simulink model "ejemplo_pendulo"  (R2018a)
settings: Solver=VariableStepAuto  StartTime=0.0  StopTime=4  MaxStep=1e-2  RelTol=1e-3
InitFcn:
  | simulacion
values from neighbouring files (symbols this model uses):
  Xe = [0 0]    [simulacion_pendulo.m]
  Xini = [0.8 0]    [simulacion_pendulo.m]
  Xinil = Xini-Xe    [simulacion_pendulo.m]
libraries: simulink x1
settings Model: Creator=cmparedes  LastModifiedBy=carma

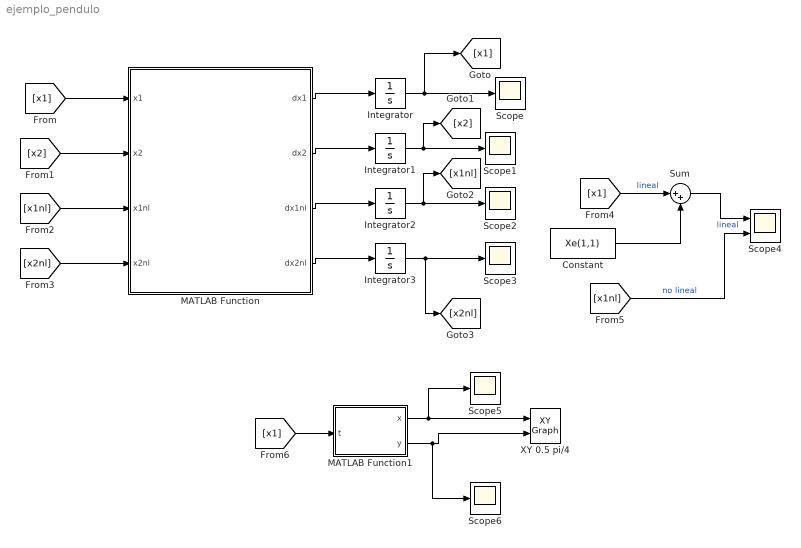
== system ejemplo_pendulo ==
  Constant : Constant  Value=Xe(1,1)
  Integrator : Integrator  InitialCondition=Xinil(1,1)
  Integrator1 : Integrator  InitialCondition=Xinil(1,2)
  Integrator2 : Integrator  InitialCondition=Xini(1,1)
  Integrator3 : Integrator  InitialCondition=Xini(1,2)
  MATLAB Function : MATLAB Function  TreatAsAtomicUnit=on
  MATLAB Function1 : MATLAB Function  TreatAsAtomicUnit=on
  Scope{,1..3,5..6} (6 alike) : Scope
  Scope4 : Scope  NumInputPorts=2
  Sum : Sum  Inputs=|++
  XY 0.5 pi/4 : simulink/Sinks/XY Graph  xmin=-0.5  xmax=0.45  ymin=-1.01  ymax=-0.92  st=-1
  wires:
  MATLAB Function/1(dx1) -> Integrator/1
  MATLAB Function/2(dx2) -> Integrator1/1
  MATLAB Function/3(dx1nl) -> Integrator2/1
  MATLAB Function/4(dx2nl) -> Integrator3/1
  Integrator/1 -> [x1], Scope/1
  Integrator1/1 -> [x2], Scope1/1
  Integrator2/1 -> [x1nl], Scope2/1
  Integrator3/1 -> [x2nl], Scope3/1
  [x1] -> MATLAB Function/1(x1)
  [x2] -> MATLAB Function/2(x2)
  [x1nl] -> MATLAB Function/3(x1nl)
  [x2nl] -> MATLAB Function/4(x2nl)
  [x1nl] -> Scope4/2  "no lineal"
  [x1] -> Sum/1  "lineal"
  Constant/1 -> Sum/2
  Sum/1 -> Scope4/1  "lineal"
  MATLAB Function1/1(x) -> Scope5/1, XY 0.5 pi/4/1
  MATLAB Function1/2(y) -> Scope6/1, XY 0.5 pi/4/2
  [x1] -> MATLAB Function1/1(t)

== matlab function ejemplo_pendulo/MATLAB Function1 ==
  data: x output; y output; t input
function [x,y] = fcn(t)
L=1;
x = L*sin(t);
y=-L*cos(t);

== matlab function ejemplo_pendulo/MATLAB Function ==
  data: dx1 output; x1 input; x2 input; dx2 output; dx1nl output; dx2nl output; x1nl input; x2nl input
function [dx1,dx2,dx1nl,dx2nl] = fcn(x1,x2,x1nl,x2nl)
x1e=0; %pi,2pi,3pi 0,261799 rad=15°
x2e=0;
g=9.8;
L=1;

dx1=x2;
dx2=(-g/L)*cos(x1e)*x1;

dx1nl=x2nl;
dx2nl=(-g/L)*sin(x1nl);
